simulink model "MultiMotor"  (Simulink 6.4)
settings: Solver=FixedStepDiscrete  StartTime=0.0  StopTime=inf  FixedStep=0.01  RelTol=1e-3
libraries: simulink x18, xpclib x4
settings Model: LastModifiedBy=Marco

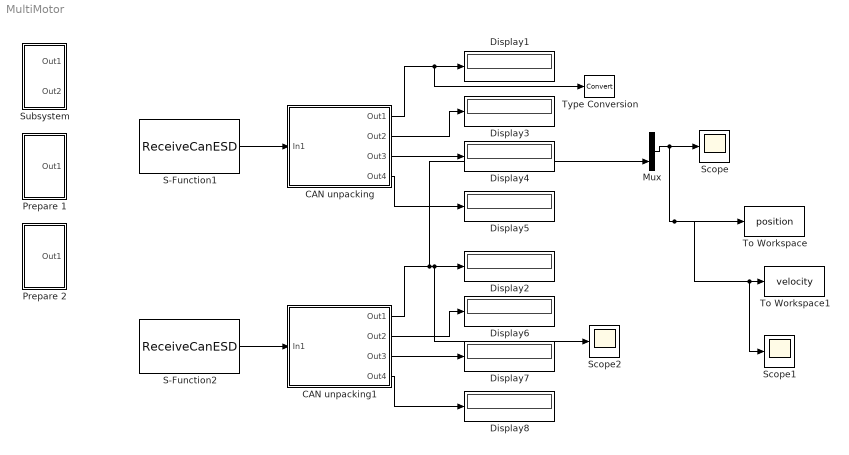
== system MultiMotor ==
  CAN unpacking : Subsystem
  CAN unpacking1 : Subsystem
  Display{1..8} (8 alike) : Display
  Mux : Mux  Inputs=2
  Prepare 1 : Subsystem
  Prepare 2 : Subsystem
  S-Function1 : S-Function  FunctionName=ReceiveCanESD  Parameters=msgID  mask{msgID=449}
      mask prompts: msgID "Message ID"
      mask Display:
      | fprintf('RECEIVE CAN\n')
      | fprintf('\nID %d',msgID);
      | port_label('output',1,'data');
  S-Function2 : S-Function  FunctionName=ReceiveCanESD  Parameters=msgID  mask{msgID=449}
      mask prompts: msgID "Message ID"
      mask Display:
      | fprintf('RECEIVE CAN\n')
      | fprintf('\nID %d',msgID);
      | port_label('output',1,'data');
  Scope : Scope
      settings: TimeRange=30  YMin=-1  YMax=1
  Scope1 : Scope
      settings: YMin=-250000  YMax=250000
  Scope2 : Scope
      settings: YMin=-1  YMax=1  SaveName=ScopeData2
  Subsystem : Subsystem
  To Workspace : ToWorkspace  VariableName=position  SampleTime=-1  SaveFormat=Structure
  To Workspace1 : ToWorkspace  VariableName=velocity  SampleTime=-1  SaveFormat=Structure
  Type Conversion : DataTypeConversion
  wires:
  CAN unpacking/1(Out1) -> Display1/1, Type Conversion/1
  CAN unpacking/2(Out2) -> Display3/1
  CAN unpacking/3(Out3) -> Display4/1
  CAN unpacking/4(Out4) -> Display5/1
  S-Function1/1 -> CAN unpacking/1(In1)
  Mux/1 -> Scope/1, To Workspace/1, To Workspace1/1, Scope1/1
  CAN unpacking1/1(Out1) -> Display2/1, Scope2/1, Mux/2
  CAN unpacking1/2(Out2) -> Display6/1
  CAN unpacking1/3(Out3) -> Display7/1
  CAN unpacking1/4(Out4) -> Display8/1
  S-Function2/1 -> CAN unpacking1/1(In1)

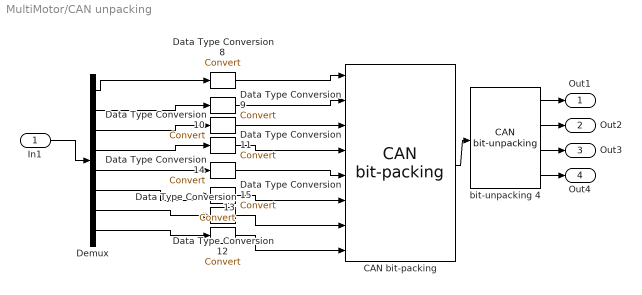
== system MultiMotor/CAN unpacking ==
  In1 : Inport
  " bit-unpacking 4" : xpclib/CAN/Utilities/CAN bit-unpacking   bitpatterns={ [0:15] [16:31] [32:47] [48:63]}  dtypes={ 'uint16' 'uint16' 'uint16' 'uint16'}
  "CAN bit-packing " : xpclib/CAN/Utilities/CAN bit-packing   bitpatterns={ [0:7] [8:15] [16:23] [24:31] [32:39] [40:47] [48:55] [56:63] }
  Data Type Conversion{8..15} (8 alike) : DataTypeConversion  OutDataTypeMode=uint8
  Demux : Demux  Outputs=8
  Out1 : Outport
  Out2 : Outport  Port=2
  Out3 : Outport  Port=3
  Out4 : Outport  Port=4
  wires:
  " bit-unpacking 4"/4 -> Out4/1
  " bit-unpacking 4"/3 -> Out3/1
  In1/1 -> Demux/1
  " bit-unpacking 4"/2 -> Out2/1
  " bit-unpacking 4"/1 -> Out1/1
  Demux/8 -> Data Type Conversion13/1
  Demux/7 -> Data Type Conversion12/1
  Demux/6 -> Data Type Conversion15/1
  Demux/5 -> Data Type Conversion14/1
  Demux/4 -> Data Type Conversion11/1
  Demux/3 -> Data Type Conversion10/1
  Demux/2 -> Data Type Conversion9/1
  Demux/1 -> Data Type Conversion8/1
  Data Type Conversion13/1 -> "CAN bit-packing "/8
  Data Type Conversion12/1 -> "CAN bit-packing "/7
  Data Type Conversion15/1 -> "CAN bit-packing "/6
  Data Type Conversion14/1 -> "CAN bit-packing "/5
  Data Type Conversion11/1 -> "CAN bit-packing "/4
  Data Type Conversion10/1 -> "CAN bit-packing "/3
  Data Type Conversion9/1 -> "CAN bit-packing "/2
  Data Type Conversion8/1 -> "CAN bit-packing "/1
  "CAN bit-packing "/1 -> " bit-unpacking 4"/1

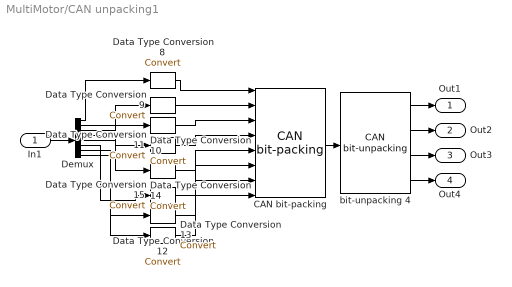
== system MultiMotor/CAN unpacking1 ==
  In1 : Inport
  " bit-unpacking 4" : xpclib/CAN/Utilities/CAN bit-unpacking   bitpatterns={ [0:15] [16:31] [32:47] [48:63]}  dtypes={ 'uint16' 'uint16' 'uint16' 'uint16'}
  "CAN bit-packing " : xpclib/CAN/Utilities/CAN bit-packing   bitpatterns={ [0:7] [8:15] [16:23] [24:31] [32:39] [40:47] [48:55] [56:63] }
  Data Type Conversion{8..15} (8 alike) : DataTypeConversion  OutDataTypeMode=uint8
  Demux : Demux  Outputs=8
  Out1 : Outport
  Out2 : Outport  Port=2
  Out3 : Outport  Port=3
  Out4 : Outport  Port=4
  wires:
  "CAN bit-packing "/1 -> " bit-unpacking 4"/1
  Data Type Conversion8/1 -> "CAN bit-packing "/1
  Data Type Conversion9/1 -> "CAN bit-packing "/2
  Data Type Conversion10/1 -> "CAN bit-packing "/3
  Data Type Conversion11/1 -> "CAN bit-packing "/4
  Data Type Conversion14/1 -> "CAN bit-packing "/5
  Data Type Conversion15/1 -> "CAN bit-packing "/6
  Data Type Conversion12/1 -> "CAN bit-packing "/7
  Data Type Conversion13/1 -> "CAN bit-packing "/8
  Demux/1 -> Data Type Conversion8/1
  Demux/2 -> Data Type Conversion9/1
  Demux/3 -> Data Type Conversion10/1
  Demux/4 -> Data Type Conversion11/1
  Demux/5 -> Data Type Conversion14/1
  Demux/6 -> Data Type Conversion15/1
  Demux/7 -> Data Type Conversion12/1
  Demux/8 -> Data Type Conversion13/1
  " bit-unpacking 4"/1 -> Out1/1
  " bit-unpacking 4"/2 -> Out2/1
  In1/1 -> Demux/1
  " bit-unpacking 4"/3 -> Out3/1
  " bit-unpacking 4"/4 -> Out4/1

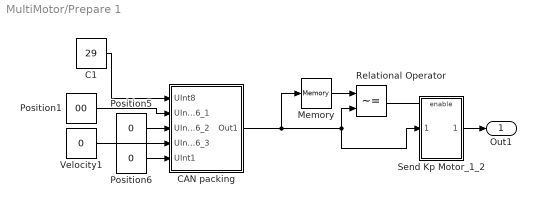
== system MultiMotor/Prepare 1 ==
  C1 : Constant  Value=29  OutDataType=sfix(16)  ConRadixGroup=Use specified scaling  OutScaling=2^0  SampleTime=inf  FramePeriod=inf
  CAN packing : Subsystem
  Memory : Memory
  Position1 : Constant  Value=00  OutDataType=sfix(16)  ConRadixGroup=Use specified scaling  OutScaling=2^0  SampleTime=inf  FramePeriod=inf
  Position5 : Constant  Value=0  OutDataType=sfix(16)  ConRadixGroup=Use specified scaling  OutScaling=2^0  SampleTime=inf  FramePeriod=inf
  Position6 : Constant  Value=0  OutDataType=sfix(16)  ConRadixGroup=Use specified scaling  OutScaling=2^0  SampleTime=inf  FramePeriod=inf
  Relational Operator : RelationalOperator  Operator=~=  LogicOutDataTypeMode=Boolean
  Send Kp Motor_1_2 : Subsystem
  Velocity1 : Constant  Value=0  OutDataType=sfix(16)  ConRadixGroup=Use specified scaling  OutScaling=2^0  SampleTime=inf  FramePeriod=inf
  Out1 : Outport
  wires:
  CAN packing/1(Out1) -> Relational Operator/2, Send Kp Motor_1_2/1(In1), Memory/1
  Position6/1 -> CAN packing/5(UInt1)
  Send Kp Motor_1_2/1(Out1) -> Out1/1
  Position5/1 -> CAN packing/3(UInt16_2)
  Velocity1/1 -> CAN packing/4(UInt16_3)
  Position1/1 -> CAN packing/2(UInt16_1)
  C1/1 -> CAN packing/1(UInt8)
  Memory/1 -> Relational Operator/1
  Relational Operator/1 -> Send Kp Motor_1_2/Enable

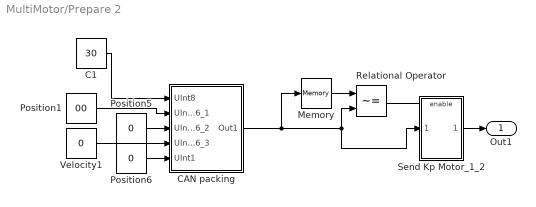
== system MultiMotor/Prepare 2 ==
  C1 : Constant  Value=30  OutDataType=sfix(16)  ConRadixGroup=Use specified scaling  OutScaling=2^0  SampleTime=inf  FramePeriod=inf
  CAN packing : Subsystem
  Memory : Memory
  Position1 : Constant  Value=00  OutDataType=sfix(16)  ConRadixGroup=Use specified scaling  OutScaling=2^0  SampleTime=inf  FramePeriod=inf
  Position5 : Constant  Value=0  OutDataType=sfix(16)  ConRadixGroup=Use specified scaling  OutScaling=2^0  SampleTime=inf  FramePeriod=inf
  Position6 : Constant  Value=0  OutDataType=sfix(16)  ConRadixGroup=Use specified scaling  OutScaling=2^0  SampleTime=inf  FramePeriod=inf
  Relational Operator : RelationalOperator  Operator=~=  LogicOutDataTypeMode=Boolean
  Send Kp Motor_1_2 : Subsystem
  Velocity1 : Constant  Value=0  OutDataType=sfix(16)  ConRadixGroup=Use specified scaling  OutScaling=2^0  SampleTime=inf  FramePeriod=inf
  Out1 : Outport
  wires:
  Relational Operator/1 -> Send Kp Motor_1_2/Enable
  Memory/1 -> Relational Operator/1
  C1/1 -> CAN packing/1(UInt8)
  Position1/1 -> CAN packing/2(UInt16_1)
  Velocity1/1 -> CAN packing/4(UInt16_3)
  Position5/1 -> CAN packing/3(UInt16_2)
  Send Kp Motor_1_2/1(Out1) -> Out1/1
  Position6/1 -> CAN packing/5(UInt1)
  CAN packing/1(Out1) -> Memory/1, Send Kp Motor_1_2/1(In1), Relational Operator/2

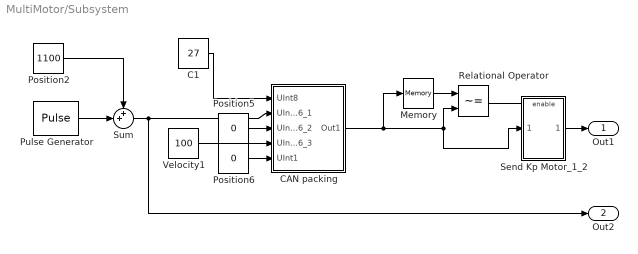
== system MultiMotor/Subsystem ==
  C1 : Constant  Value=27  OutDataType=sfix(16)  ConRadixGroup=Use specified scaling  OutScaling=2^0  SampleTime=inf  FramePeriod=inf
  CAN packing : Subsystem
  Memory : Memory
  Position2 : Constant  Value=1100  OutDataType=sfix(16)  ConRadixGroup=Use specified scaling  OutScaling=2^0  SampleTime=inf  FramePeriod=inf
  Position5 : Constant  Value=0  OutDataType=sfix(16)  ConRadixGroup=Use specified scaling  OutScaling=2^0  SampleTime=inf  FramePeriod=inf
  Position6 : Constant  Value=0  OutDataType=sfix(16)  ConRadixGroup=Use specified scaling  OutScaling=2^0  SampleTime=inf  FramePeriod=inf
  Pulse Generator : DiscretePulseGenerator  PulseType=Time based  Amplitude=1000  Period=16  PulseWidth=50
  Relational Operator : RelationalOperator  Operator=~=  LogicOutDataTypeMode=Boolean
  Send Kp Motor_1_2 : Subsystem
  Sum : Sum  Inputs=++|
  Velocity1 : Constant  Value=100  OutDataType=sfix(16)  ConRadixGroup=Use specified scaling  OutScaling=2^0  SampleTime=inf  FramePeriod=inf
  Out1 : Outport
  Out2 : Outport  Port=2
  wires:
  Relational Operator/1 -> Send Kp Motor_1_2/Enable
  Memory/1 -> Relational Operator/1
  C1/1 -> CAN packing/1(UInt8)
  Sum/1 -> CAN packing/2(UInt16_1), Out2/1
  Velocity1/1 -> CAN packing/4(UInt16_3)
  Position5/1 -> CAN packing/3(UInt16_2)
  Send Kp Motor_1_2/1(Out1) -> Out1/1
  Position6/1 -> CAN packing/5(UInt1)
  CAN packing/1(Out1) -> Memory/1, Send Kp Motor_1_2/1(In1), Relational Operator/2
  Pulse Generator/1 -> Sum/2
  Position2/1 -> Sum/1

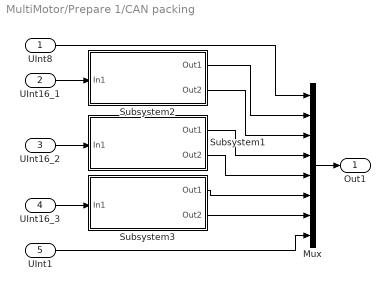
== system MultiMotor/Prepare 1/CAN packing ==
  UInt8 : Inport
  UInt16_1 : Inport  Port=2
  UInt16_2 : Inport  Port=3
  UInt16_3 : Inport  Port=4
  UInt1 : Inport  Port=5
  Mux : Mux  Inputs=8
  Subsystem1 : Subsystem
  Subsystem2 : Subsystem
  Subsystem3 : Subsystem
  Out1 : Outport
  wires:
  UInt1/1 -> Mux/8
  Subsystem3/2(Out2) -> Mux/7
  Subsystem3/1(Out1) -> Mux/6
  UInt16_3/1 -> Subsystem3/1(In1)
  Subsystem1/2(Out2) -> Mux/5
  Subsystem1/1(Out1) -> Mux/4
  UInt16_2/1 -> Subsystem1/1(In1)
  Subsystem2/1(Out1) -> Mux/2
  UInt16_1/1 -> Subsystem2/1(In1)
  Subsystem2/2(Out2) -> Mux/3
  UInt8/1 -> Mux/1
  Mux/1 -> Out1/1

== system MultiMotor/Prepare 1/Send Kp Motor_1_2 ==
  In1 : Inport
  Enable : EnablePort
  GO_1_2 : S-Function  FunctionName=SendCanESD  Parameters=(baudrate-1),msgid,length  mask{baudrate=1000 Kbits/s, msgid=12, length=5}
      mask prompts: msgid "Message ID"; length "Message Length"
      mask StyleString: popup(1000 Kbits/s|500  Kbits/s),edit,edit
      mask Display:
      | fprintf('SEND CAN\n')
      | fprintf('\nID %d',msgid);
      | port_label('input',1,'message');
      | color('red');port_label('output',1,'status');
  Out1 : Outport
  wires:
  GO_1_2/1 -> Out1/1
  In1/1 -> GO_1_2/1

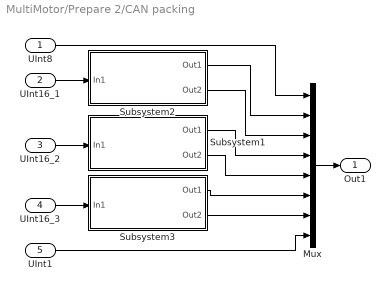
== system MultiMotor/Prepare 2/CAN packing ==
  UInt8 : Inport
  UInt16_1 : Inport  Port=2
  UInt16_2 : Inport  Port=3
  UInt16_3 : Inport  Port=4
  UInt1 : Inport  Port=5
  Mux : Mux  Inputs=8
  Subsystem1 : Subsystem
  Subsystem2 : Subsystem
  Subsystem3 : Subsystem
  Out1 : Outport
  wires:
  Mux/1 -> Out1/1
  UInt8/1 -> Mux/1
  Subsystem2/2(Out2) -> Mux/3
  UInt16_1/1 -> Subsystem2/1(In1)
  Subsystem2/1(Out1) -> Mux/2
  UInt16_2/1 -> Subsystem1/1(In1)
  Subsystem1/1(Out1) -> Mux/4
  Subsystem1/2(Out2) -> Mux/5
  UInt16_3/1 -> Subsystem3/1(In1)
  Subsystem3/1(Out1) -> Mux/6
  Subsystem3/2(Out2) -> Mux/7
  UInt1/1 -> Mux/8

== system MultiMotor/Prepare 2/Send Kp Motor_1_2 ==
  In1 : Inport
  Enable : EnablePort
  GO_1_2 : S-Function  FunctionName=SendCanESD  Parameters=(baudrate-1),msgid,length  mask{baudrate=1000 Kbits/s, msgid=12, length=5}
      mask prompts: msgid "Message ID"; length "Message Length"
      mask StyleString: popup(1000 Kbits/s|500  Kbits/s),edit,edit
      mask Display:
      | fprintf('SEND CAN\n')
      | fprintf('\nID %d',msgid);
      | port_label('input',1,'message');
      | color('red');port_label('output',1,'status');
  Out1 : Outport
  wires:
  In1/1 -> GO_1_2/1
  GO_1_2/1 -> Out1/1

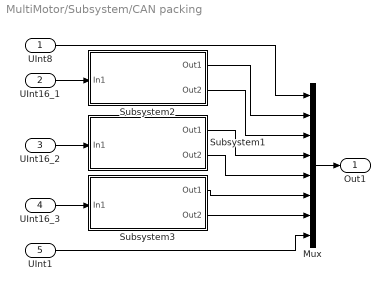
== system MultiMotor/Subsystem/CAN packing ==
  UInt8 : Inport
  UInt16_1 : Inport  Port=2
  UInt16_2 : Inport  Port=3
  UInt16_3 : Inport  Port=4
  UInt1 : Inport  Port=5
  Mux : Mux  Inputs=8
  Subsystem1 : Subsystem
  Subsystem2 : Subsystem
  Subsystem3 : Subsystem
  Out1 : Outport
  wires:
  Mux/1 -> Out1/1
  UInt8/1 -> Mux/1
  Subsystem2/2(Out2) -> Mux/3
  UInt16_1/1 -> Subsystem2/1(In1)
  Subsystem2/1(Out1) -> Mux/2
  UInt16_2/1 -> Subsystem1/1(In1)
  Subsystem1/1(Out1) -> Mux/4
  Subsystem1/2(Out2) -> Mux/5
  UInt16_3/1 -> Subsystem3/1(In1)
  Subsystem3/1(Out1) -> Mux/6
  Subsystem3/2(Out2) -> Mux/7
  UInt1/1 -> Mux/8

== system MultiMotor/Subsystem/Send Kp Motor_1_2 ==
  In1 : Inport
  Enable : EnablePort
  GO_1_2 : S-Function  FunctionName=SendCanESD  Parameters=(baudrate-1),msgid,length  mask{baudrate=1000 Kbits/s, msgid=13, length=7}
      mask prompts: msgid "Message ID"; length "Message Length"
      mask StyleString: popup(1000 Kbits/s|500  Kbits/s),edit,edit
      mask Display:
      | fprintf('SEND CAN\n')
      | fprintf('\nID %d',msgid);
      | port_label('input',1,'message');
      | color('red');port_label('output',1,'status');
  Out1 : Outport
  wires:
  In1/1 -> GO_1_2/1
  GO_1_2/1 -> Out1/1

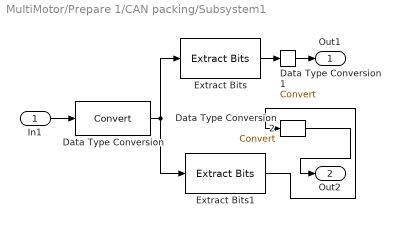
== system MultiMotor/Prepare 1/CAN packing/Subsystem1 ==
  In1 : Inport
  Data Type Conversion : DataTypeConversion  OutDataTypeMode=uint16
  Data Type Conversion1 : DataTypeConversion  OutDataTypeMode=double
  Data Type Conversion2 : DataTypeConversion  OutDataTypeMode=double
  Extract Bits : simulink/Logic and Bit Operations/Extract Bits  SystemSampleTime=-1  bitsToExtract=Range of bits  numBits=8  bitIdxRange=[0 7]  outScalingMode=Treat bit field as an integer
  Extract Bits1 : simulink/Logic and Bit Operations/Extract Bits  SystemSampleTime=-1  bitsToExtract=Range of bits  numBits=8  bitIdxRange=[8 15]  outScalingMode=Treat bit field as an integer
  Out1 : Outport
  Out2 : Outport  Port=2
  wires:
  Extract Bits1/1 -> Data Type Conversion2/1
  Data Type Conversion2/1 -> Out2/1
  Data Type Conversion1/1 -> Out1/1
  In1/1 -> Data Type Conversion/1
  Extract Bits/1 -> Data Type Conversion1/1
  Data Type Conversion/1 -> Extract Bits/1, Extract Bits1/1

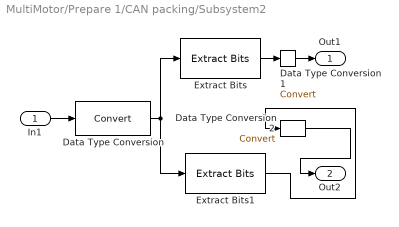
== system MultiMotor/Prepare 1/CAN packing/Subsystem2 ==
  In1 : Inport
  Data Type Conversion : DataTypeConversion  OutDataTypeMode=uint16
  Data Type Conversion1 : DataTypeConversion  OutDataTypeMode=double
  Data Type Conversion2 : DataTypeConversion  OutDataTypeMode=double
  Extract Bits : simulink/Logic and Bit Operations/Extract Bits  SystemSampleTime=-1  bitsToExtract=Range of bits  numBits=8  bitIdxRange=[0 7]  outScalingMode=Treat bit field as an integer
  Extract Bits1 : simulink/Logic and Bit Operations/Extract Bits  SystemSampleTime=-1  bitsToExtract=Range of bits  numBits=8  bitIdxRange=[8 15]  outScalingMode=Treat bit field as an integer
  Out1 : Outport
  Out2 : Outport  Port=2
  wires:
  Data Type Conversion/1 -> Extract Bits1/1, Extract Bits/1
  Extract Bits/1 -> Data Type Conversion1/1
  In1/1 -> Data Type Conversion/1
  Data Type Conversion1/1 -> Out1/1
  Data Type Conversion2/1 -> Out2/1
  Extract Bits1/1 -> Data Type Conversion2/1

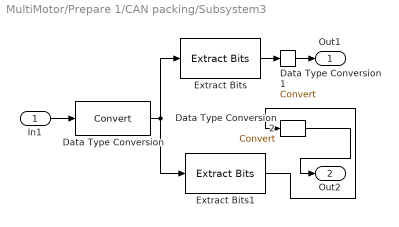
== system MultiMotor/Prepare 1/CAN packing/Subsystem3 ==
  In1 : Inport
  Data Type Conversion : DataTypeConversion  OutDataTypeMode=uint16
  Data Type Conversion1 : DataTypeConversion  OutDataTypeMode=double
  Data Type Conversion2 : DataTypeConversion  OutDataTypeMode=double
  Extract Bits : simulink/Logic and Bit Operations/Extract Bits  SystemSampleTime=-1  bitsToExtract=Range of bits  numBits=8  bitIdxRange=[0 7]  outScalingMode=Treat bit field as an integer
  Extract Bits1 : simulink/Logic and Bit Operations/Extract Bits  SystemSampleTime=-1  bitsToExtract=Range of bits  numBits=8  bitIdxRange=[8 15]  outScalingMode=Treat bit field as an integer
  Out1 : Outport
  Out2 : Outport  Port=2
  wires:
  Data Type Conversion/1 -> Extract Bits1/1, Extract Bits/1
  Extract Bits/1 -> Data Type Conversion1/1
  In1/1 -> Data Type Conversion/1
  Data Type Conversion1/1 -> Out1/1
  Data Type Conversion2/1 -> Out2/1
  Extract Bits1/1 -> Data Type Conversion2/1

== system MultiMotor/Prepare 2/CAN packing/Subsystem1 ==
  In1 : Inport
  Data Type Conversion : DataTypeConversion  OutDataTypeMode=uint16
  Data Type Conversion1 : DataTypeConversion  OutDataTypeMode=double
  Data Type Conversion2 : DataTypeConversion  OutDataTypeMode=double
  Extract Bits : simulink/Logic and Bit Operations/Extract Bits  SystemSampleTime=-1  bitsToExtract=Range of bits  numBits=8  bitIdxRange=[0 7]  outScalingMode=Treat bit field as an integer
  Extract Bits1 : simulink/Logic and Bit Operations/Extract Bits  SystemSampleTime=-1  bitsToExtract=Range of bits  numBits=8  bitIdxRange=[8 15]  outScalingMode=Treat bit field as an integer
  Out1 : Outport
  Out2 : Outport  Port=2
  wires:
  Data Type Conversion/1 -> Extract Bits1/1, Extract Bits/1
  Extract Bits/1 -> Data Type Conversion1/1
  In1/1 -> Data Type Conversion/1
  Data Type Conversion1/1 -> Out1/1
  Data Type Conversion2/1 -> Out2/1
  Extract Bits1/1 -> Data Type Conversion2/1

== system MultiMotor/Prepare 2/CAN packing/Subsystem2 ==
  In1 : Inport
  Data Type Conversion : DataTypeConversion  OutDataTypeMode=uint16
  Data Type Conversion1 : DataTypeConversion  OutDataTypeMode=double
  Data Type Conversion2 : DataTypeConversion  OutDataTypeMode=double
  Extract Bits : simulink/Logic and Bit Operations/Extract Bits  SystemSampleTime=-1  bitsToExtract=Range of bits  numBits=8  bitIdxRange=[0 7]  outScalingMode=Treat bit field as an integer
  Extract Bits1 : simulink/Logic and Bit Operations/Extract Bits  SystemSampleTime=-1  bitsToExtract=Range of bits  numBits=8  bitIdxRange=[8 15]  outScalingMode=Treat bit field as an integer
  Out1 : Outport
  Out2 : Outport  Port=2
  wires:
  Extract Bits1/1 -> Data Type Conversion2/1
  Data Type Conversion2/1 -> Out2/1
  Data Type Conversion1/1 -> Out1/1
  In1/1 -> Data Type Conversion/1
  Extract Bits/1 -> Data Type Conversion1/1
  Data Type Conversion/1 -> Extract Bits/1, Extract Bits1/1

== system MultiMotor/Prepare 2/CAN packing/Subsystem3 ==
  In1 : Inport
  Data Type Conversion : DataTypeConversion  OutDataTypeMode=uint16
  Data Type Conversion1 : DataTypeConversion  OutDataTypeMode=double
  Data Type Conversion2 : DataTypeConversion  OutDataTypeMode=double
  Extract Bits : simulink/Logic and Bit Operations/Extract Bits  SystemSampleTime=-1  bitsToExtract=Range of bits  numBits=8  bitIdxRange=[0 7]  outScalingMode=Treat bit field as an integer
  Extract Bits1 : simulink/Logic and Bit Operations/Extract Bits  SystemSampleTime=-1  bitsToExtract=Range of bits  numBits=8  bitIdxRange=[8 15]  outScalingMode=Treat bit field as an integer
  Out1 : Outport
  Out2 : Outport  Port=2
  wires:
  Extract Bits1/1 -> Data Type Conversion2/1
  Data Type Conversion2/1 -> Out2/1
  Data Type Conversion1/1 -> Out1/1
  In1/1 -> Data Type Conversion/1
  Extract Bits/1 -> Data Type Conversion1/1
  Data Type Conversion/1 -> Extract Bits/1, Extract Bits1/1

== system MultiMotor/Subsystem/CAN packing/Subsystem1 ==
  In1 : Inport
  Data Type Conversion : DataTypeConversion  OutDataTypeMode=uint16
  Data Type Conversion1 : DataTypeConversion  OutDataTypeMode=double
  Data Type Conversion2 : DataTypeConversion  OutDataTypeMode=double
  Extract Bits : simulink/Logic and Bit Operations/Extract Bits  SystemSampleTime=-1  bitsToExtract=Range of bits  numBits=8  bitIdxRange=[0 7]  outScalingMode=Treat bit field as an integer
  Extract Bits1 : simulink/Logic and Bit Operations/Extract Bits  SystemSampleTime=-1  bitsToExtract=Range of bits  numBits=8  bitIdxRange=[8 15]  outScalingMode=Treat bit field as an integer
  Out1 : Outport
  Out2 : Outport  Port=2
  wires:
  Data Type Conversion/1 -> Extract Bits1/1, Extract Bits/1
  Extract Bits/1 -> Data Type Conversion1/1
  In1/1 -> Data Type Conversion/1
  Data Type Conversion1/1 -> Out1/1
  Data Type Conversion2/1 -> Out2/1
  Extract Bits1/1 -> Data Type Conversion2/1

== system MultiMotor/Subsystem/CAN packing/Subsystem2 ==
  In1 : Inport
  Data Type Conversion : DataTypeConversion  OutDataTypeMode=uint16
  Data Type Conversion1 : DataTypeConversion  OutDataTypeMode=double
  Data Type Conversion2 : DataTypeConversion  OutDataTypeMode=double
  Extract Bits : simulink/Logic and Bit Operations/Extract Bits  SystemSampleTime=-1  bitsToExtract=Range of bits  numBits=8  bitIdxRange=[0 7]  outScalingMode=Treat bit field as an integer
  Extract Bits1 : simulink/Logic and Bit Operations/Extract Bits  SystemSampleTime=-1  bitsToExtract=Range of bits  numBits=8  bitIdxRange=[8 15]  outScalingMode=Treat bit field as an integer
  Out1 : Outport
  Out2 : Outport  Port=2
  wires:
  Extract Bits1/1 -> Data Type Conversion2/1
  Data Type Conversion2/1 -> Out2/1
  Data Type Conversion1/1 -> Out1/1
  In1/1 -> Data Type Conversion/1
  Extract Bits/1 -> Data Type Conversion1/1
  Data Type Conversion/1 -> Extract Bits/1, Extract Bits1/1

== system MultiMotor/Subsystem/CAN packing/Subsystem3 ==
  In1 : Inport
  Data Type Conversion : DataTypeConversion  OutDataTypeMode=uint16
  Data Type Conversion1 : DataTypeConversion  OutDataTypeMode=double
  Data Type Conversion2 : DataTypeConversion  OutDataTypeMode=double
  Extract Bits : simulink/Logic and Bit Operations/Extract Bits  SystemSampleTime=-1  bitsToExtract=Range of bits  numBits=8  bitIdxRange=[0 7]  outScalingMode=Treat bit field as an integer
  Extract Bits1 : simulink/Logic and Bit Operations/Extract Bits  SystemSampleTime=-1  bitsToExtract=Range of bits  numBits=8  bitIdxRange=[8 15]  outScalingMode=Treat bit field as an integer
  Out1 : Outport
  Out2 : Outport  Port=2
  wires:
  Extract Bits1/1 -> Data Type Conversion2/1
  Data Type Conversion2/1 -> Out2/1
  Data Type Conversion1/1 -> Out1/1
  In1/1 -> Data Type Conversion/1
  Extract Bits/1 -> Data Type Conversion1/1
  Data Type Conversion/1 -> Extract Bits/1, Extract Bits1/1
